simulink model "conv_droop_2Rinv"  (R2026a)
settings: Solver=ode23t  StopTime=8  MaxStep=1e-4  RelTol=1e-4
libraries: fl_lib x10, nesl_utility x7
settings Model: Creator=runzedeng  LastModifiedBy=runzedeng

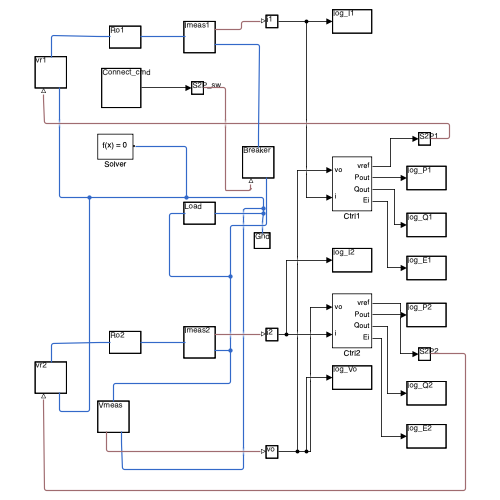
[thumbnail: Simulink's stored preview of the top-level diagram]
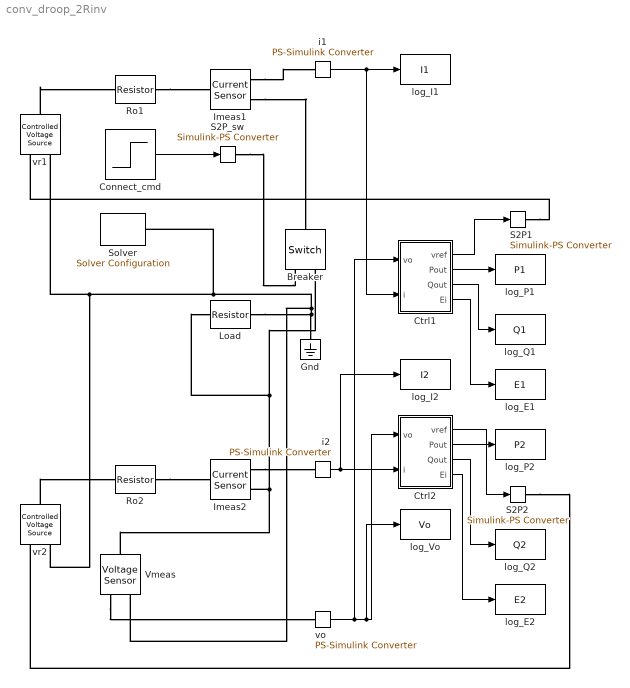
== system conv_droop_2Rinv ==
  Breaker : fl_lib/Electrical/Electrical Elements/Switch  R_closed=1e-3 Ohm  G_open=1e-4 1/Ohm  Threshold=0.5  i_specify=off  i_priority=None  i=0 A  i_nominal_specify=off  i_nominal_value=1  i_nominal_unit=A  v_specify=off  v_priority=None  v=0 V  v_nominal_specify=off  v_nominal_value=1  v_nominal_unit=V
  Connect_cmd : Step  Time=3
  Ctrl1 : Subsystem
  Ctrl2 : Subsystem
  Gnd : fl_lib/Electrical/Electrical Elements/Electrical Reference
  Imeas1 : fl_lib/Electrical/Electrical Sensors/Current Sensor
  Imeas2 : fl_lib/Electrical/Electrical Sensors/Current Sensor
  Load : fl_lib/Electrical/Electrical Elements/Resistor  R=9 Ohm  i_specify=off  i_priority=None  i=0 A  i_nominal_specify=off  i_nominal_value=1  i_nominal_unit=A  v_specify=off  v_priority=None  v=0 V  v_nominal_specify=off  v_nominal_value=1  v_nominal_unit=V
  Ro1 : fl_lib/Electrical/Electrical Elements/Resistor  R=1 Ohm  i_specify=off  i_priority=None  i=0 A  i_nominal_specify=off  i_nominal_value=1  i_nominal_unit=A  v_specify=off  v_priority=None  v=0 V  v_nominal_specify=off  v_nominal_value=1  v_nominal_unit=V
  Ro2 : fl_lib/Electrical/Electrical Elements/Resistor  R=1 Ohm  i_specify=off  i_priority=None  i=0 A  i_nominal_specify=off  i_nominal_value=1  i_nominal_unit=A  v_specify=off  v_priority=None  v=0 V  v_nominal_specify=off  v_nominal_value=1  v_nominal_unit=V
  S2P1 : nesl_utility/Simulink-PS Converter  PhysicalDomain=network_engine_domain  SubClassName=ps_input  LeftPortType=input  RightPortType=output  PseudoPeriodic=off  Frequencies=[]  NoiseDistribution=none  NoiseParameters=[]  Unit=1  AffineConversion=off  FilteringAndDerivatives=provide  SimscapeFilterOrder=1  InputFilterTimeConstant=0.001  UdotUserProvided=0
  S2P2 : nesl_utility/Simulink-PS Converter  PhysicalDomain=network_engine_domain  SubClassName=ps_input  LeftPortType=input  RightPortType=output  PseudoPeriodic=off  Frequencies=[]  NoiseDistribution=none  NoiseParameters=[]  Unit=1  AffineConversion=off  FilteringAndDerivatives=provide  SimscapeFilterOrder=1  InputFilterTimeConstant=0.001  UdotUserProvided=0
  S2P_sw : nesl_utility/Simulink-PS Converter  PhysicalDomain=network_engine_domain  SubClassName=ps_input  LeftPortType=input  RightPortType=output  PseudoPeriodic=off  Frequencies=[]  NoiseDistribution=none  NoiseParameters=[]  Unit=1  AffineConversion=off  FilteringAndDerivatives=provide  SimscapeFilterOrder=1  InputFilterTimeConstant=0.001  UdotUserProvided=0
  Solver : nesl_utility/Solver Configuration  PhysicalDomain=network_engine_domain  SubClassName=solver  LeftPortType=input  RightPortType=generic  Tones=[]  Harmonics=[]  SimulateNoise=off  Profile=off  UseLocalSampling=off  EnableSwitchedLinearOptims=on  FrequencyDomain=off  UseCCode=off  RelTol=0.001  AbsTol=0.001  MinStep=1e-09  ToWorkspace=off  RevertToSquareIcSolve=off  NumHomotopyIterations=100  PhasorMode=off  PhasorModeNumHarmonics=1  ConsistencySolver=NEWTON_XTOL_AFTER_FTOL  CanonicalOrdering=CANONICAL  OptimizeIntermediates=OPTIMIZED  IndexReductionMethod=DerivativeReplacement  DoDC=off  ResidualTolerance=1e-09  ConsistencyTolSource=GLOBAL  ConsistencyAbsTol=0.001  ConsistencyRelTol=0.001  ConsistencyTolFactor=0.001  UseLocalSolver=off  LocalSolverChoice=NE_BACKWARD_EULER_ADVANCER  ResolveIndetEquations=on  FunctionEvalNumThread=1  LocalSolverSampleTime=0.001  DoFixedCost=off  MaxNonlinIter=3  MaxModeIter=2  ComputeImpulses=off  ImpulseIterations=2  LinearAlgebra=auto  LinearAlgebraNumThread=0  EquationFormulation=NE_TIME_EF  DelaysMemoryBudget=1024  AutomaticFiltering=on  FilteringTimeConstant=0.001  PartitionStorageMethod=AS_NEEDED  PartitionMemoryBudget=1024  PartitionMethod=ROBUST  MultibodyUseLocalSolver=off  MultibodyLocalSolverChoice=ODE1  MultibodyLocalSolverSampleTime=0.001
  Vmeas : fl_lib/Electrical/Electrical Sensors/Voltage Sensor
  i1 : nesl_utility/PS-Simulink Converter  PhysicalDomain=network_engine_domain  SubClassName=ps_output  LeftPortType=input  RightPortType=output  PseudoPeriodic=off  Frequencies=[]  VectorFormat=inherit  Unit=inherit  AffineConversion=off
  i2 : nesl_utility/PS-Simulink Converter  PhysicalDomain=network_engine_domain  SubClassName=ps_output  LeftPortType=input  RightPortType=output  PseudoPeriodic=off  Frequencies=[]  VectorFormat=inherit  Unit=inherit  AffineConversion=off
  log_E1 : ToWorkspace  VariableName=E1  SaveFormat=Timeseries
  log_E2 : ToWorkspace  VariableName=E2  SaveFormat=Timeseries
  log_I1 : ToWorkspace  VariableName=I1  SaveFormat=Timeseries
  log_I2 : ToWorkspace  VariableName=I2  SaveFormat=Timeseries
  log_P1 : ToWorkspace  VariableName=P1  SaveFormat=Timeseries
  log_P2 : ToWorkspace  VariableName=P2  SaveFormat=Timeseries
  log_Q1 : ToWorkspace  VariableName=Q1  SaveFormat=Timeseries
  log_Q2 : ToWorkspace  VariableName=Q2  SaveFormat=Timeseries
  log_Vo : ToWorkspace  VariableName=Vo  SaveFormat=Timeseries
  vo : nesl_utility/PS-Simulink Converter  PhysicalDomain=network_engine_domain  SubClassName=ps_output  LeftPortType=input  RightPortType=output  PseudoPeriodic=off  Frequencies=[]  VectorFormat=inherit  Unit=inherit  AffineConversion=off
  vr1 : fl_lib/Electrical/Electrical Sources/Controlled Voltage Source
  vr2 : fl_lib/Electrical/Electrical Sources/Controlled Voltage Source
  wires:
  Ctrl2/1(vref) -> S2P2/1
  Ctrl1/4(Ei) -> log_E1/1
  Ctrl1/2(Pout) -> log_P1/1
  Ctrl1/1(vref) -> S2P1/1
  vo/1 -> log_Vo/1, Ctrl2/1(vo), Ctrl1/1(vo)
  Ctrl2/4(Ei) -> log_E2/1
  Ctrl1/3(Qout) -> log_Q1/1
  Ctrl2/3(Qout) -> log_Q2/1
  Ctrl2/2(Pout) -> log_P2/1
  Connect_cmd/1 -> S2P_sw/1
  i1/1 -> log_I1/1, Ctrl1/2(i)
  i2/1 -> log_I2/1, Ctrl2/2(i)
  connections:
  S2P1/RConn1 -- vr1/RConn1
  vr2/LConn1 -- Ro2/LConn1
  Ro2/RConn1 -- Imeas2/LConn1
  Imeas2/RConn1 -- i2/LConn1
  Load/RConn1 -- vr2/RConn2 -- vr1/RConn2 -- Solver/RConn1 -- Vmeas/RConn2 -- Gnd/LConn1
  S2P_sw/RConn1 -- Breaker/RConn1
  Imeas1/RConn2 -- Breaker/LConn1
  S2P2/RConn1 -- vr2/RConn1
  Vmeas/LConn1 -- Breaker/RConn2 -- Load/LConn1 -- Imeas2/RConn2
  vr1/LConn1 -- Ro1/LConn1
  Imeas1/RConn1 -- i1/LConn1
  Ro1/RConn1 -- Imeas1/LConn1
  Vmeas/RConn1 -- vo/LConn1

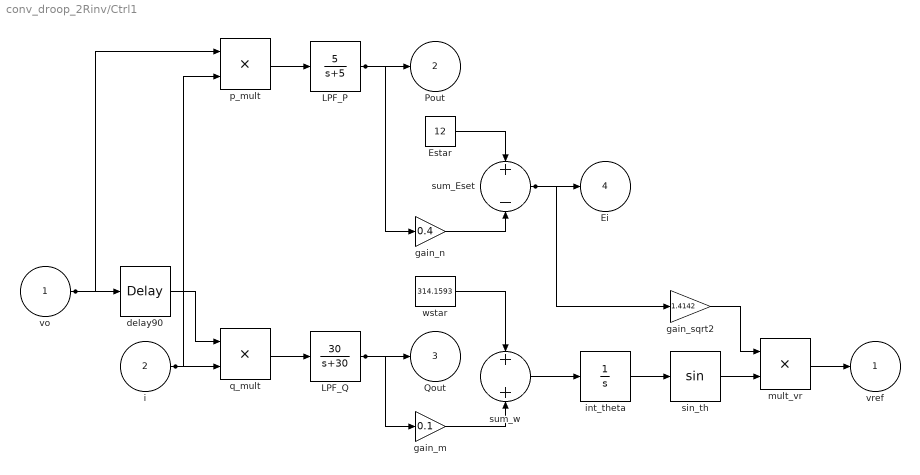
== system conv_droop_2Rinv/Ctrl1 ==
  vo : Inport
  i : Inport  Port=2
  Estar : Constant  Value=12
  LPF_P : TransferFcn  Numerator=5  Denominator=[1 5]
  LPF_Q : TransferFcn  Numerator=30  Denominator=[1 30]
  delay90 : TransportDelay  DelayTime=0.005
  gain_m : Gain  Gain=0.1
  gain_n : Gain  Gain=0.4
  gain_sqrt2 : Gain  Gain=1.4142
  int_theta : Integrator
  mult_vr : Product
  p_mult : Product
  q_mult : Product
  sin_th : Trigonometry
  sum_Eset : Sum  Inputs=+-
  sum_w : Sum
  wstar : Constant  Value=314.1593
  vref : Outport
  Pout : Outport  Port=2
  Qout : Outport  Port=3
  Ei : Outport  Port=4
  wires:
  mult_vr/1 -> vref/1
  gain_sqrt2/1 -> mult_vr/1
  sin_th/1 -> mult_vr/2
  gain_n/1 -> sum_Eset/2
  Estar/1 -> sum_Eset/1
  wstar/1 -> sum_w/1
  int_theta/1 -> sin_th/1
  q_mult/1 -> LPF_Q/1
  vo/1 -> delay90/1, p_mult/1
  LPF_P/1 -> Pout/1, gain_n/1
  sum_Eset/1 -> Ei/1, gain_sqrt2/1
  gain_m/1 -> sum_w/2
  p_mult/1 -> LPF_P/1
  i/1 -> q_mult/2, p_mult/2
  delay90/1 -> q_mult/1
  sum_w/1 -> int_theta/1
  LPF_Q/1 -> Qout/1, gain_m/1

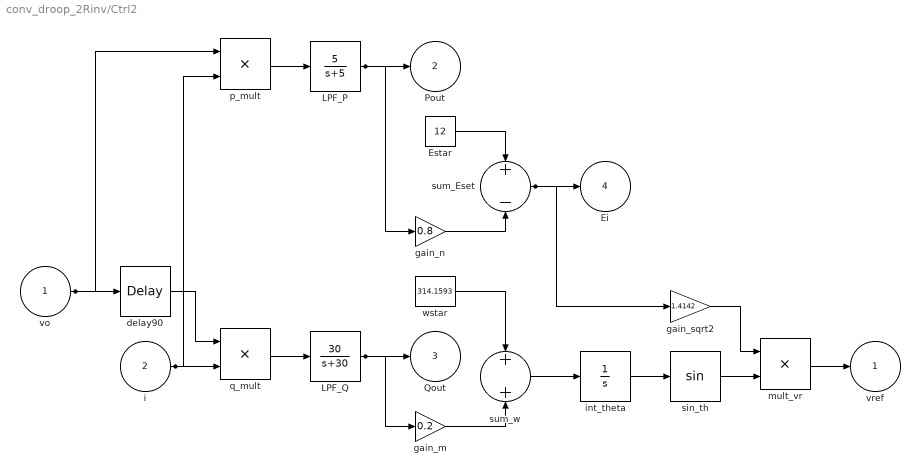
== system conv_droop_2Rinv/Ctrl2 ==
  vo : Inport
  i : Inport  Port=2
  Estar : Constant  Value=12
  LPF_P : TransferFcn  Numerator=5  Denominator=[1 5]
  LPF_Q : TransferFcn  Numerator=30  Denominator=[1 30]
  delay90 : TransportDelay  DelayTime=0.005
  gain_m : Gain  Gain=0.2
  gain_n : Gain  Gain=0.8
  gain_sqrt2 : Gain  Gain=1.4142
  int_theta : Integrator
  mult_vr : Product
  p_mult : Product
  q_mult : Product
  sin_th : Trigonometry
  sum_Eset : Sum  Inputs=+-
  sum_w : Sum
  wstar : Constant  Value=314.1593
  vref : Outport
  Pout : Outport  Port=2
  Qout : Outport  Port=3
  Ei : Outport  Port=4
  wires:
  mult_vr/1 -> vref/1
  sin_th/1 -> mult_vr/2
  int_theta/1 -> sin_th/1
  sum_w/1 -> int_theta/1
  gain_m/1 -> sum_w/2
  wstar/1 -> sum_w/1
  gain_n/1 -> sum_Eset/2
  LPF_P/1 -> Pout/1, gain_n/1
  Estar/1 -> sum_Eset/1
  LPF_Q/1 -> Qout/1, gain_m/1
  i/1 -> q_mult/2, p_mult/2
  q_mult/1 -> LPF_Q/1
  gain_sqrt2/1 -> mult_vr/1
  vo/1 -> delay90/1, p_mult/1
  p_mult/1 -> LPF_P/1
  sum_Eset/1 -> Ei/1, gain_sqrt2/1
  delay90/1 -> q_mult/1
